simulink model "castor_NO-VALIDO"  (R2021b)
settings: Solver=VariableStepAuto  StartTime=0.0  StopTime=10.0  MaxStep=0.01  RelTol=1e-3
settings Model: Creator=Daniel  LastModifiedBy=Daniel

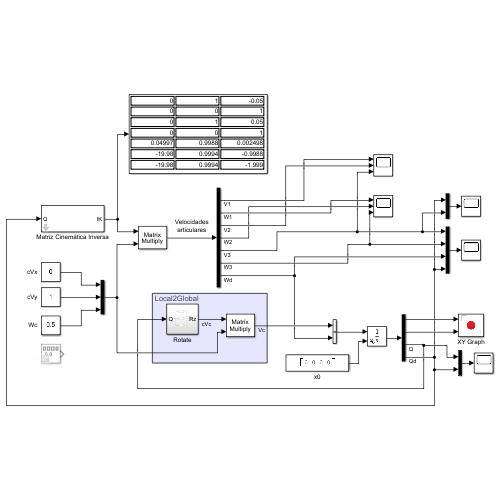
[thumbnail: Simulink's stored preview of the top-level diagram]
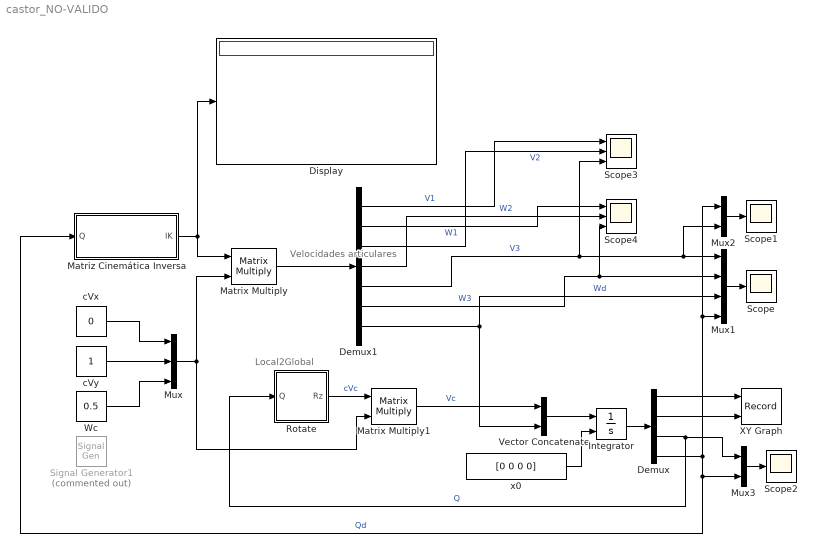
== system castor_NO-VALIDO ==
  note: Local2Global
  note: Velocidades
      | articulares
  Demux : Demux
  Demux1 : Demux  Outputs=7
  Display : Display
  Integrator : Integrator  InitialConditionSource=external
  Matrix Multiply : Product  Multiplication=Matrix(*)
  Matrix Multiply1 : Product  Multiplication=Matrix(*)
  Matriz Cinemática Inversa : Subsystem  mask{d1=0.05, d2=0.05, d3=0.05, d4=0.05}
      mask prompts: d1 "Traction Wheel1 Offset"; d2 "Traction Wheel2 Offset"; d3 "Steering Offset"; d4 "Steering Length"
  Mux : Mux  Inputs=3
  Mux1 : Mux
  Mux2 : Mux  Inputs=2
  Mux3 : Mux  Inputs=2
  Rotate : Subsystem
  Scope : Scope
  Scope1 : Scope
  Scope2 : Scope
  Scope3 : Scope  NumInputPorts=3
  Scope4 : Scope  NumInputPorts=3
  Signal Generator1 : SignalGenerator  Commented=on  WaveForm=square  Amplitude=2  Frequency=0.32
  Vector Concatenate : Concatenate
  Wc : Constant  Value=0.5
  XY Graph : Record  FileSettingsInternal="{\"entries\":[{\"content\":{\"excelSettings\":{\"content\":{},\"type\":\"Streamout.ExcelSettings\"}},\"type\":\"Streamout.FileSettingStorage\",\"uuid\":\"dd344777-611f-45d0-ac3e-c9eee2e57a05\"}],\"packageUris\":[\"http://schema.mathworks.com/mf0/streamout_blocks/R2020a\"],\"version\":\"1.0\"}"  Layout=[1 1]  SignalsInternal="{\"entries\":[{\"content\":{\"signals\":[{\"content\":{\"blockPath\":[\"castor/XY Graph\"],\"channel\":[],\"dimensions\":[1,1],\"domain\":\"castor/XY Graph\",\"lineColor\":\"#a2142f\",\"plots\":[1],\"port\":1,\"sid\":[\"\"],\"signalID\":1427,\"signalName\":\"Demux:1\"},\"type\":\"RecordBlkView.Signal\",\"uuid\":\"fad05bde-8ebd-4e7d-8796-017d9cfad601\"},{\"content\":{\"blockPath\":[\"castor/XY Graph\"],\"channel\":[],\"dimensions\":[1,1],\"domain\":\"castor/XY Graph\",\"lineColor\":\"#139fff\",\"plots\":[1],\"port\":2,\"sid\":[\"\"],\"signalID\":1431,\"signalName\":\"Demux:2\"},\"type\":\"RecordBlkView.Signal\",\"uuid\":\"6d3f59db-4d86-4bfc-8fb6-285c0dcac875\"}]},\"type\":\"RecordBlkView.InputSignals\",\"uuid\":\"16be6882-cbfa-4022-a035-b77a753fe0bd\"}],\"packageUris\":[\"http://schema.mathworks.com/mf0/streamout_blocks/R2020a\"],\"version\":\"1.0\"}"  VisualizationBindings="{\"xyplotplugin\":{\"info\":[{\"series\":[{\"bindingParametersList\":[{\"parameter\":\"X-Axis\",\"signalID\":1427,\"signalName\":\"Demux:1\"},{\"parameter\":\"Y-Axis\",\"signalID\":1431,\"signalName\":\"Demux:2\"}],\"seriesID\":5348}],\"subplotID\":1}]}}"  CompatibilityTag=XY
  cVx : Constant  Value=0
  cVy : Constant
  x0 : Constant  Value=[0 0 0 0]  VectorParams1D=off  SampleTime=-1
  wires:
  cVy/1 -> Mux/2
  cVx/1 -> Mux/1
  Matriz Cinemática Inversa/1(IK) -> Matrix Multiply/1, Display/1
  Mux/1 -> Matrix Multiply/2, Matrix Multiply1/2
  Vector Concatenate/1 -> Integrator/1
  Integrator/1 -> Demux/1
  Demux/1 -> XY Graph/1
  Demux/2 -> XY Graph/2
  Demux/4 -> Mux2/1, Mux1/4, Mux3/2, Matriz Cinemática Inversa/1(Q)  "Qd"
  Matrix Multiply1/1 -> Vector Concatenate/1  "Vc"
  Matrix Multiply/1 -> Demux1/1
  Demux1/7 -> Mux1/3, Vector Concatenate/2  "Wd"
  Demux1/6 -> Scope4/3, Mux1/2  "W3"
  Demux1/5 -> Scope3/3, Mux2/2, Mux1/1  "V3"
  Mux1/1 -> Scope/1
  x0/1 -> Integrator/2
  Rotate/1(Rz) -> Matrix Multiply1/1  "cVc"
  Demux/3 -> Mux3/1, Rotate/1(Q)  "Q"
  Mux2/1 -> Scope1/1
  Mux3/1 -> Scope2/1
  Wc/1 -> Mux/3
  Demux1/1 -> Scope3/1  "V1"
  Demux1/3 -> Scope3/2  "V2"
  Demux1/2 -> Scope4/1  "W1"
  Demux1/4 -> Scope4/2  "W2"

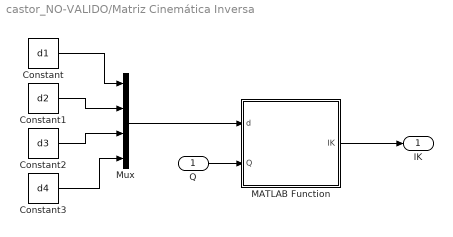
== system castor_NO-VALIDO/Matriz Cinemática Inversa ==
  Q : Inport
  Constant : Constant  Value=d1
  Constant1 : Constant  Value=d2
  Constant2 : Constant  Value=d3
  Constant3 : Constant  Value=d4
  MATLAB Function : MATLAB Function  TreatAsAtomicUnit=on
  Mux : Mux
  IK : Outport
  wires:
  Q/1 -> MATLAB Function/2(Q)
  MATLAB Function/1(IK) -> IK/1
  Constant1/1 -> Mux/2
  Constant2/1 -> Mux/3
  Constant/1 -> Mux/1
  Constant3/1 -> Mux/4
  Mux/1 -> MATLAB Function/1(d)

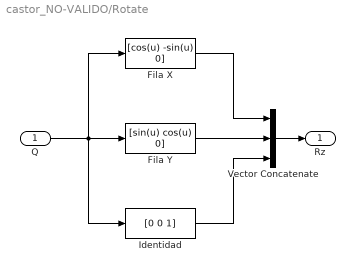
== system castor_NO-VALIDO/Rotate ==
  Q : Inport
  Fila X : MATLABFcn  MATLABFcn=[cos(u) -sin(u) 0]  OutputDimensions=[1 3]  Output1D=off
  Fila Y : MATLABFcn  MATLABFcn=[sin(u) cos(u) 0]  OutputDimensions=[1 3]  Output1D=off
  Identidad : MATLABFcn  MATLABFcn=[0 0 1]  OutputDimensions=[1 3]  Output1D=off
  Vector Concatenate : Concatenate  NumInputs=3  Mode=Multidimensional array
  Rz : Outport
  wires:
  Q/1 -> Identidad/1, Fila Y/1, Fila X/1
  Vector Concatenate/1 -> Rz/1
  Fila Y/1 -> Vector Concatenate/2
  Fila X/1 -> Vector Concatenate/1
  Identidad/1 -> Vector Concatenate/3

== matlab function castor_NO-VALIDO/Matriz Cinemática Inversa/MATLAB Function ==
  data: d input; IK output; Q input
function IK = fcn(d,Q)

    J1 = [0 0; 1 d(1); 0 1];
    J2 = [0 0; 1 -d(2); 0 1];
    J3 = [-sin(Q) -d(4)*cos(Q)-d(3) d(3); cos(Q) -d(4)*sin(Q) 0; 0 1 -1];
    
    % Creación de las matrices A y Jacobiana
    A=[eye(3); eye(3); eye(3)];
    B=[J1 zeros(3,2) zeros(3,3); zeros(3,2) J2 zeros(3,3); zeros(3,2) zeros(3,2) J3];

    IK = inv(B'*B)*B'*A;

end
